simulink model "TIController_SpeedgoatInterface_"  (R2023b)
settings: Solver=FixedStepAuto  StartTime=0.0  StopTime=Inf  FixedStep=0.001  RelTol=1e-3
settings Model: DVDesignModelName=SimulationMain  DVExtractedSubsystem=TI Controller (Speedgoat Interface)  Creator=rodri  LastModifiedBy=rodri
settings SolverCC: ConcurrentTasks=on  PositivePriorityOrder=on
settings OptimizationCC: BlockReduction=off  OptimizeBlockIOStorage=off
settings DebuggingCC: TasksWithSamePriorityMsg=none  FrameProcessingCompatibilityMsg=none
settings HardwareCC: ProdBitPerLong=64  ProdLongLongMode=on  ProdHWDeviceType=Intel->x86-64 (Linux 64)
settings ModelReferenceCC: ModelReferenceNumInstancesAllowed=Single
settings RTWCC: Description=Simulink Real-Time  SystemTargetFile=slrealtime.tlc  TemplateMakefile=slrealtime_default_tmf  Toolchain=Simulink Real-Time Toolchain  BuildConfiguration=Faster Runs  CodeExecutionProfiling=on  TargetLang=C++

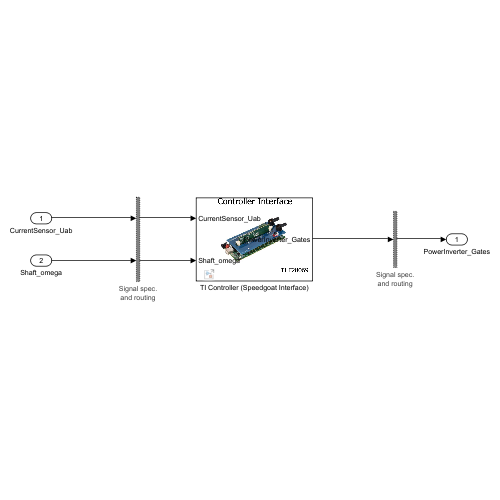
[thumbnail: Simulink's stored preview of the top-level diagram]
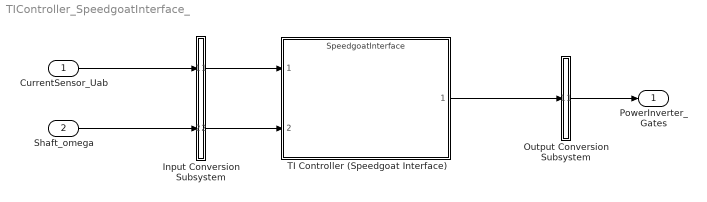
== system TIController_SpeedgoatInterface_ ==
  CurrentSensor_Uab : Inport  OutDataTypeStr=double  PortDimensions=[2]  SampleTime=0.001  Interpolate=off
  Shaft_omega : Inport  Port=2  OutDataTypeStr=double  PortDimensions=[1]  SampleTime=0.001  Interpolate=off
  Input Conversion Subsystem : Subsystem  Tag=__SLT_ICS__  Description=|
      | Signal spec.
      | and routing
      settings: AttributesFormatString=%<Description>
  Output Conversion Subsystem : Subsystem  Tag=__SLT_OCS__  Description=|
      | Signal spec.
      | and routing
      settings: AttributesFormatString=%<Description>
  TI Controller (Speedgoat Interface) : ModelReference  ModelNameDialog=SpeedgoatInterface.slx  SimulationMode=Normal  ModelReferenceVersion=1.10
      mask Display: image('controller_interface.svg');
  PowerInverter_Gates : Outport
  wires:
  CurrentSensor_Uab/1 -> Input Conversion Subsystem/1(Inport_1)
  Shaft_omega/1 -> Input Conversion Subsystem/2(Inport_2)
  Output Conversion Subsystem/1(Outport_1) -> PowerInverter_Gates/1
  Input Conversion Subsystem/1(Outport_1) -> TI Controller (Speedgoat Interface)/1
  Input Conversion Subsystem/2(Outport_2) -> TI Controller (Speedgoat Interface)/2
  TI Controller (Speedgoat Interface)/1 -> Output Conversion Subsystem/1(Inport_1)

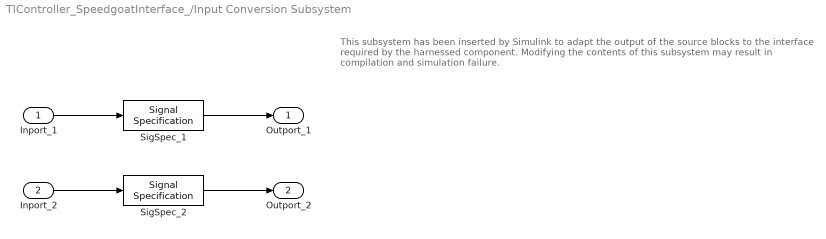
== system TIController_SpeedgoatInterface_/Input Conversion Subsystem ==
  note: This subsystem has been inserted by Simulink to adapt the output of the source blocks to the interface required by the harnessed component.
      |  Modifying the contents of this subsystem may result in compilation and simulation failure.
  Inport_1 : Inport
  Inport_2 : Inport  Port=2
  SigSpec_1 : SignalSpecification  OutDataTypeStr=double  Dimensions=[2]  SampleTime=0.001
  SigSpec_2 : SignalSpecification  OutDataTypeStr=double  Dimensions=[1]  SampleTime=0.001
  Outport_1 : Outport
  Outport_2 : Outport  Port=2
  wires:
  SigSpec_1/1 -> Outport_1/1
  Inport_1/1 -> SigSpec_1/1
  SigSpec_2/1 -> Outport_2/1
  Inport_2/1 -> SigSpec_2/1

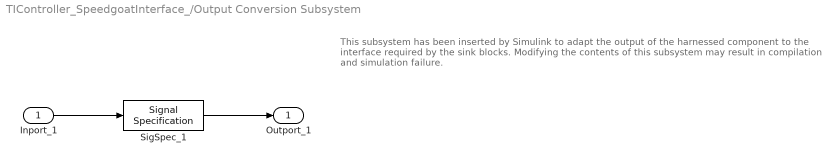
== system TIController_SpeedgoatInterface_/Output Conversion Subsystem ==
  note: This subsystem has been inserted by Simulink to adapt the output of the harnessed component to the interface required by the sink blocks.
      |  Modifying the contents of this subsystem may result in compilation and simulation failure.
  Inport_1 : Inport
  SigSpec_1 : SignalSpecification  OutDataTypeStr=double  Dimensions=[6]  SampleTime=0.001
  Outport_1 : Outport
  wires:
  Inport_1/1 -> SigSpec_1/1
  SigSpec_1/1 -> Outport_1/1
